simulink model "guidance_fuzzy_alt"  (R2017b)
settings: Solver=FixedStepDiscrete  StartTime=0.0  StopTime=inf  FixedStep=0.01  RelTol=1e-3
model workspace (MAT data in the model file):
  SL_ROS_VariableLengthArrays_MaxSizes.CommonInfo.ArrayTruncateAction = 'EmitWarning'
  SL_ROS_VariableLengthArrays_MaxSizes.MsgTypeMap = containers.Map
  SL_ROS_VariableLengthArrays_MaxSizes.MsgTypeMap.serialization.keys = {'sensor_msgs/Image'}
  SL_ROS_VariableLengthArrays_MaxSizes.MsgTypeMap.serialization.values{1}(1).PropertyName = 'Encoding'
  SL_ROS_VariableLengthArrays_MaxSizes.MsgTypeMap.serialization.values{1}(1).DataType = 'uint8'
  SL_ROS_VariableLengthArrays_MaxSizes.MsgTypeMap.serialization.values{1}(1).MaxLength = 128
  SL_ROS_VariableLengthArrays_MaxSizes.MsgTypeMap.serialization.values{1}(2).PropertyName = 'Data'
  SL_ROS_VariableLengthArrays_MaxSizes.MsgTypeMap.serialization.values{1}(2).DataType = 'uint8'
  SL_ROS_VariableLengthArrays_MaxSizes.MsgTypeMap.serialization.values{1}(2).MaxLength = 921600
  SL_ROS_VariableLengthArrays_MaxSizes.MsgTypeMap.serialization.uniformity = 0
  SL_ROS_VariableLengthArrays_MaxSizes.MsgTypeMap.serialization.keyType = 'char'
  SL_ROS_VariableLengthArrays_MaxSizes.MsgTypeMap.serialization.valueType = 'any'
undefined symbols (not defined in the file): Data, Data_SL_Info
libraries: dspstat3 x14, robotlib x10, simulink_extras x7, simulink x4, dspswit3 x1
(part 1 of 2)
settings Model: SimulationMode=external  Creator=a  LastModifiedBy=Alien
settings OptimizationCC: MaxStackSize=64
settings DebuggingCC: ParameterTunabilityLossMsg=error
settings HardwareCC: ProdBitPerPointer=32  ProdBitPerSizeT=32  ProdBitPerPtrDiffT=32  ProdLargestAtomicInteger=Long  ProdLargestAtomicFloat=Double  ProdWordSize=32  ProdHWDeviceType=ARM Compatible->ARM Cortex
settings SFSimCC: MATLABDynamicMemAlloc=off
settings RTWCC: SystemTargetFile=ert.tlc  HardwareBoard=Robot Operating System (ROS)  TemplateMakefile=ert_default_tmf  GenerateReport=on  Toolchain=Catkin  IncludeHyperlinkInReport=on  LaunchReport=on  TargetLang=C++  GenerateTraceInfo=on  GenerateTraceReport=on  GenerateTraceReportSl=on  GenerateTraceReportSf=on  GenerateTraceReportEml=on
settings CodeAppCC: ForceParamTrailComments=on  IgnoreCustomStorageClasses=off  OperatorAnnotations=on  SimulinkDataObjDesc=on  SFDataObjDesc=on  MATLABFcnDesc=on  InsertBlockDesc=on  StateflowObjectComments=on  MATLABSourceComments=on
settings ERTTargetCC: MultiwordLength=2048  ExtMode=on  ExtModeMexArgs='192.168.2.2' 0 17725
settings SimscapeCC: SimscapeNormalizeSystem=off

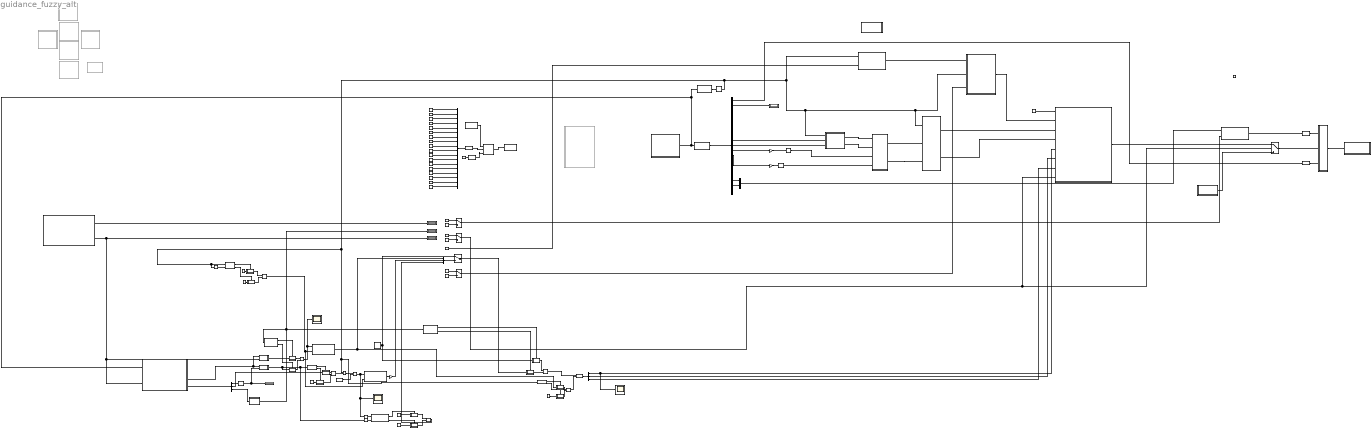
== system guidance_fuzzy_alt ==
  note: Subsystem
  Abs6 : Abs
  Abs7 : Abs
  Assignment : Assignment  DiagnosticForDimensions=Warning  IndexOptions=Index vector (dialog)  Indices=1  OutputSizes=1
  Blank Message : robotlib/Blank Message  SourceLibraryInfo=This block requires Robotics System Toolbox  messageType=std_msgs/UInt8MultiArray  SampleTime=inf
      settings: SourceProductBaseCode=RO
  Bus Assignment : BusAssignment  AssignedSignals=Data,Data_SL_Info.CurrentLength
  Constant : Constant  Value=[0 0 0]
  Constant1 : Constant  Value=18:128
  Constant2 : Constant  Value=0
  Constant3 : Constant  Value=17
  Constant4 : Constant
  Constant5 : Constant  Value=0
  Constant6 : Constant  Value=0
  "Count_QRcodes " : Display
  Course : Display
  Data Store Memory : DataStoreMemory  DataStoreName=kill  ReadBeforeWriteMsg=warning  WriteAfterWriteMsg=warning  WriteAfterReadMsg=warning  ShowAdditionalParam=off
  Data Type Conversion18 : DataTypeConversion  OutDataTypeStr=uint8
  Data Type Conversion19 : DataTypeConversion  OutDataTypeStr=uint32
  Data Type Conversion3 : DataTypeConversion  OutDataTypeStr=single
  Data Type Conversion4 : DataTypeConversion  OutDataTypeStr=single
  DataChangeTimer : Subsystem
  Demux : Demux  Outputs=19
  Demux1 : Demux  Outputs=3
  Demux6 : Demux  Outputs=3
  Discrete PID Controller : simulink/Continuous/PID Controller  Controller=PID  TimeDomain=Discrete-time  SampleTime=-1  IntegratorMethod=Forward Euler  FilterMethod=Forward Euler  Form=Parallel  UseFilter=on  ControllerParametersSource=internal  P=0.4  I=0.001  D=0  N=100  InitialConditionSource=internal  InitialConditionForIntegrator=0  InitialConditionForFilter=0  ExternalReset=either  LimitOutput=on  UpperSaturationLimit=10  LowerSaturationLimit=-10  LinearizeAsGain=off  AntiWindupMode=none  Kb=1  TrackingMode=off  Kt=1  PParamMin=[]  PParamMax=[]  IParamMin=[]  IParamMax=[]  DParamMin=[]  DParamMax=[]  NParamMin=[]  NParamMax=[]  KbParamMin=[]  KbParamMax=[]  KtParamMin=[]  KtParamMax=[]  POutMin=[]  POutMax=[]  IOutMin=[]  IOutMax=[]  DOutMin=[]  DOutMax=[]  NOutMin=[]  NOutMax=[]  KbOutMin=[]  KbOutMax=[]  KtOutMin=[]  KtOutMax=[]  IntegratorOutMin=[]  IntegratorOutMax=[]  FilterOutMin=[]  FilterOutMax=[]  SumOutMin=[]  SumOutMax=[]  SumI1OutMin=[]  SumI1OutMax=[]  SumI2OutMin=[]  SumI2OutMax=[]  SumI3OutMin=[]  SumI3OutMax=[]  SumDOutMin=[]  SumDOutMax=[]  SaturationOutMin=[]  SaturationOutMax=[]  IntegratorContinuousStateAttributes=''  IntegratorStateMustResolveToSignalObject=off  IntegratorRTWStateStorageClass=Auto  FilterContinuousStateAttributes=''  FilterStateMustResolveToSignalObject=off  FilterRTWStateStorageClass=Auto  DifferentiatorICPrevScaledInput=0  DifferentiatorOutMin=[]  DifferentiatorOutMax=[]  InitialConditionSetting=State (most efficient)  FilterDiffOutCoefMin=[]  FilterDiffOutCoefMax=[]  SumDenOutMin=[]  SumDenOutMax=[]  SumNumOutMin=[]  SumNumOutMax=[]  ReciprocalOutMin=[]  ReciprocalOutMax=[]  DivideOutMin=[]  DivideOutMax=[]  TunerSelectOption=Transfer Function Based (PID Tuner App)
  Discrete PID Controller1 : simulink/Continuous/PID Controller  Controller=PID  TimeDomain=Discrete-time  SampleTime=-1  IntegratorMethod=Forward Euler  FilterMethod=Forward Euler  Form=Parallel  UseFilter=on  ControllerParametersSource=internal  P=0.2  I=0  D=0  N=100  InitialConditionSource=internal  InitialConditionForIntegrator=0  InitialConditionForFilter=0  ExternalReset=either  LimitOutput=on  UpperSaturationLimit=0.5  LowerSaturationLimit=-0.5  LinearizeAsGain=off  AntiWindupMode=none  Kb=1  TrackingMode=off  Kt=1  PParamMin=[]  PParamMax=[]  IParamMin=[]  IParamMax=[]  DParamMin=[]  DParamMax=[]  NParamMin=[]  NParamMax=[]  KbParamMin=[]  KbParamMax=[]  KtParamMin=[]  KtParamMax=[]  POutMin=[]  POutMax=[]  IOutMin=[]  IOutMax=[]  DOutMin=[]  DOutMax=[]  NOutMin=[]  NOutMax=[]  KbOutMin=[]  KbOutMax=[]  KtOutMin=[]  KtOutMax=[]  IntegratorOutMin=[]  IntegratorOutMax=[]  FilterOutMin=[]  FilterOutMax=[]  SumOutMin=[]  SumOutMax=[]  SumI1OutMin=[]  SumI1OutMax=[]  SumI2OutMin=[]  SumI2OutMax=[]  SumI3OutMin=[]  SumI3OutMax=[]  SumDOutMin=[]  SumDOutMax=[]  SaturationOutMin=[]  SaturationOutMax=[]  IntegratorContinuousStateAttributes=''  IntegratorStateMustResolveToSignalObject=off  IntegratorRTWStateStorageClass=Auto  FilterContinuousStateAttributes=''  FilterStateMustResolveToSignalObject=off  FilterRTWStateStorageClass=Auto  DifferentiatorICPrevScaledInput=0  DifferentiatorOutMin=[]  DifferentiatorOutMax=[]  InitialConditionSetting=State (most efficient)  FilterDiffOutCoefMin=[]  FilterDiffOutCoefMax=[]  SumDenOutMin=[]  SumDenOutMax=[]  SumNumOutMin=[]  SumNumOutMax=[]  ReciprocalOutMin=[]  ReciprocalOutMax=[]  DivideOutMin=[]  DivideOutMax=[]  TunerSelectOption=Transfer Function Based (PID Tuner App)
  Display10 : Display
  Divide : Product  Inputs=*/
  Gain2 : Gain  Gain=-1
  If : If  NumInputs=2  IfExpression=u1 < 0.15 & u2 < 15
  If Action Subsystem : Subsystem  TreatAsAtomicUnit=on
  If Action Subsystem1 : Subsystem  TreatAsAtomicUnit=on
  If Action Subsystem10 : Subsystem  TreatAsAtomicUnit=on
  If Action Subsystem11 : Subsystem  TreatAsAtomicUnit=on
  If Action Subsystem2 : Subsystem  TreatAsAtomicUnit=on
  If Action Subsystem3 : Subsystem  TreatAsAtomicUnit=on
  If Action Subsystem4 : Subsystem  TreatAsAtomicUnit=on
  If Action Subsystem5 : Subsystem  TreatAsAtomicUnit=on
  If Action Subsystem6 : Subsystem  TreatAsAtomicUnit=on
  If Action Subsystem7 : Subsystem  TreatAsAtomicUnit=on
  If Action Subsystem8 : Subsystem  TreatAsAtomicUnit=on
  If Action Subsystem9 : Subsystem  TreatAsAtomicUnit=on
  If1 : If  IfExpression=u1 < 10
  If11 : If  IfExpression=u1 > 2
  If2 : If  IfExpression=u1 > 2
  If3 : If  NumInputs=2  IfExpression=u1 > 0.2 & u2<0.2
  If4 : If  IfExpression=u1 > 0.2
  Manual Switch : ManualSwitch
  Memory : Memory
  Merge{,1..5} (6 alike) : Merge
  Moving Average : dspstat3/Moving Average  Method=Sliding window  SpecifyWindowLength=on  WindowLength=30  ForgettingFactor=0.9  SimulateUsing=Code generation
  Mux3 : Mux  Inputs=3
  Mux4 : Mux  Inputs=2
  Mux8 : Mux  Inputs=18
  P Moving Average : dspstat3/Moving Average  Method=Sliding window  SpecifyWindowLength=on  WindowLength=35  ForgettingFactor=0.9  SimulateUsing=Code generation
  Product : Product
  Publish : robotlib/Publish  SourceLibraryInfo=This block requires Robotics System Toolbox  topicSource=Specify your own  topic=/quadrotor_1/params  messageType=std_msgs/UInt8MultiArray  messageQueueLength=1
      settings: SourceProductBaseCode=RO
  Push Button : Subsystem  Commented=on  DialogController=hmiCreateDDGDialog  IsWebBlock=on  mask(MWDashboardBlock){webBlockId=dc87a16a-ce0b-429d-b1f9-30aaadb48afa, webBlockType=pushbutton, ShowInLibBrwoser=on, ShowInitialText=on, HMISrcModelName=guidance_fuzzy_alt}
      mask prompts: webBlockId "WebBlock Id"; webBlockType "WebBlock Type"; HMISrcModelName "Source Model"
      mask help: SimulinkHMI:dialogs:PushButtonDialogDesc
      mask Help: helpview([docroot '/mapfiles/simulink.map'], 'hmi_push_button')
      mask Display:
      | model = bdroot(gcb);
      | if strcmp(get_param(model,'BlockDiagramType'), 'library')
      |     image([(matlabroot) '/toolbox/simulink/hmi/icons/PushButton.png']);
      | end
  Push Button1 : Subsystem  Commented=on  DialogController=hmiCreateDDGDialog  IsWebBlock=on  mask(MWDashboardBlock){webBlockId=24acbbf4-6844-475c-bdac-e05cc7a3fcf0, webBlockType=pushbutton, ShowInLibBrwoser=on, ShowInitialText=on, HMISrcModelName=guidance_fuzzy_alt}
      mask prompts: webBlockId "WebBlock Id"; webBlockType "WebBlock Type"; HMISrcModelName "Source Model"
      mask help: SimulinkHMI:dialogs:PushButtonDialogDesc
      mask Help: helpview([docroot '/mapfiles/simulink.map'], 'hmi_push_button')
      mask Display:
      | model = bdroot(gcb);
      | if strcmp(get_param(model,'BlockDiagramType'), 'library')
      |     image([(matlabroot) '/toolbox/simulink/hmi/icons/PushButton.png']);
      | end
  Push Button2 : Subsystem  Commented=on  DialogController=hmiCreateDDGDialog  IsWebBlock=on  mask(MWDashboardBlock){webBlockId=70708495-3a8b-4125-b41c-8b8a1e915131, webBlockType=pushbutton, ShowInLibBrwoser=on, ShowInitialText=on, HMISrcModelName=guidance_fuzzy_alt}
      mask prompts: webBlockId "WebBlock Id"; webBlockType "WebBlock Type"; HMISrcModelName "Source Model"
      mask help: SimulinkHMI:dialogs:PushButtonDialogDesc
      mask Help: helpview([docroot '/mapfiles/simulink.map'], 'hmi_push_button')
      mask Display:
      | model = bdroot(gcb);
      | if strcmp(get_param(model,'BlockDiagramType'), 'library')
      |     image([(matlabroot) '/toolbox/simulink/hmi/icons/PushButton.png']);
      | end
  Push Button3 : Subsystem  Commented=on  DialogController=hmiCreateDDGDialog  IsWebBlock=on  mask(MWDashboardBlock){webBlockId=ffc355a9-f3f0-46c2-899e-34688d84451c, webBlockType=pushbutton, ShowInLibBrwoser=on, ShowInitialText=on, HMISrcModelName=guidance_fuzzy_alt}
      mask prompts: webBlockId "WebBlock Id"; webBlockType "WebBlock Type"; HMISrcModelName "Source Model"
      mask help: SimulinkHMI:dialogs:PushButtonDialogDesc
      mask Help: helpview([docroot '/mapfiles/simulink.map'], 'hmi_push_button')
      mask Display:
      | model = bdroot(gcb);
      | if strcmp(get_param(model,'BlockDiagramType'), 'library')
      |     image([(matlabroot) '/toolbox/simulink/hmi/icons/PushButton.png']);
      | end
  Push Button4 : Subsystem  Commented=on  DialogController=hmiCreateDDGDialog  IsWebBlock=on  mask(MWDashboardBlock){webBlockId=54db0c4f-5f86-4b76-bb6a-5be3d8ea16bb, webBlockType=pushbutton, ShowInLibBrwoser=on, ShowInitialText=on, HMISrcModelName=guidance_fuzzy_alt}
      mask prompts: webBlockId "WebBlock Id"; webBlockType "WebBlock Type"; HMISrcModelName "Source Model"
      mask help: SimulinkHMI:dialogs:PushButtonDialogDesc
      mask Help: helpview([docroot '/mapfiles/simulink.map'], 'hmi_push_button')
      mask Display:
      | model = bdroot(gcb);
      | if strcmp(get_param(model,'BlockDiagramType'), 'library')
      |     image([(matlabroot) '/toolbox/simulink/hmi/icons/PushButton.png']);
      | end
  Push Button5 : Subsystem  Commented=on  DialogController=hmiCreateDDGDialog  IsWebBlock=on  mask(MWDashboardBlock){webBlockId=7ebe0749-6d9c-49fd-940b-537e52e049aa, webBlockType=pushbutton, ShowInLibBrwoser=on, ShowInitialText=on, HMISrcModelName=guidance_fuzzy_alt}
      mask prompts: webBlockId "WebBlock Id"; webBlockType "WebBlock Type"; HMISrcModelName "Source Model"
      mask help: SimulinkHMI:dialogs:PushButtonDialogDesc
      mask Help: helpview([docroot '/mapfiles/simulink.map'], 'hmi_push_button')
      mask Display:
      | model = bdroot(gcb);
      | if strcmp(get_param(model,'BlockDiagramType'), 'library')
      |     image([(matlabroot) '/toolbox/simulink/hmi/icons/PushButton.png']);
      | end
  Q Moving Average : dspstat3/Moving Average  Method=Sliding window  SpecifyWindowLength=on  WindowLength=35  ForgettingFactor=0.9  SimulateUsing=Code generation
  Scope1 : Scope
  Scope2 : Scope
  Scope3 : Scope
  Selector : Selector  InputPortWidth=26  IndexOptions=Index vector (dialog)  Indices=[17:26 4 5 6 11 12 13 1:3]  OutputSizes=1
  Selector1 : Selector  InputPortWidth=26  IndexOptions=Index vector (dialog)  Indices=[7]  OutputSizes=1
  Slider Switch : Subsystem  Commented=on  DialogController=hmiCreateDDGDialog  IsWebBlock=on  mask(MWDashboardBlock){webBlockId=a556c2db-78b9-4d66-bd76-d44e139280cd, webBlockType=sliderswitch, ShowInLibBrowser=on, ShowInitialText=on, HMISrcModelName=guidance_fuzzy_alt}
      mask prompts: webBlockId "WebBlock Id"; webBlockType "WebBlock Type"; HMISrcModelName "Source Model"
      mask help: SimulinkHMI:dialogs:SwitchDialogDesc
      mask Help: helpview([docroot '/mapfiles/simulink.map'], 'hmi_slider_switch')
      mask Display:
      | if strcmp(get_param(bdroot(gcb),'BlockDiagramType'), 'library')
      |     image([(matlabroot) '/toolbox/simulink/hmi/icons/SliderSwitch.png']);
      | end
  Sonar Moving Average : dspstat3/Moving Average  Method=Sliding window  SpecifyWindowLength=on  WindowLength=5  ForgettingFactor=0.9  SimulateUsing=Code generation
  Subsystem : Subsystem
  Subsystem2 : Subsystem
  Subsystem5 : Subsystem
  Subsystem6 : Subsystem
  Switch : Switch  Criteria=u2 > Threshold
  "TIme_From Last_line " : Display
  approx_poly_eppsilon_coef : Constant  Value=2
  arm_switch : ManualSwitch
  aspect_ratio_max : Constant  Value=100
  aspect_ratio_min : Constant  Value=3
  attitude_failsafe : Subsystem
  camera_trigonometric_factor(m/pix) : Constant  Value=342.85
  check_arm_status : Subsystem
  command_input : Subsystem  Commented=on
  command_output : Subsystem
  compensate_angular_velocity_effect_on_of : Subsystem
  corrupt_max_area : Constant  Value=60
  "dark_max_b " : Constant  Value=90
  dark_max_g : Constant  Value=90
  dark_max_r : Constant  Value=90
  dark_min_b : Constant  Value=0
  dark_min_g : Constant  Value=0
  dark_min_r : Constant  Value=0
  "data_input " : Subsystem
  land : ManualSwitch
  manual_control : Subsystem  mask{throttle=0.0, roll=0, pitch=0, yaw=0, mode=2}
  manual_throttle : Subsystem  mask{th=90}
  max_diviation : Constant  Value=40
  mode : Constant  Value=2
  movement_velocity : Constant  Value=0.1
  movement_velocity1 : Constant  Value=0
  one : Constant
  one1 : Constant
  one2 : Constant
  optimize_error_psi(deg)1 : Subsystem
  optimize_error_psi(deg)3 : Subsystem
  p gain : Gain  Gain=3.1415 / 180.0
  pixel_per_sec_to_m_per_sec : Subsystem
  q gain : Gain  Gain=3.1415 / 180.0
  radio_command_frame_rate : Display
  take_off_switch : ManualSwitch
  throttle_handler_climb_mode : Subsystem
  velocity_control : Subsystem
  white_max_b : Constant  Value=255
  white_max_g : Constant  Value=255
  white_max_r : Constant  Value=255
  white_min_b : Constant  Value=120
  white_min_g : Constant  Value=120
  white_min_r : Constant  Value=120
  z_des : Constant
  zero : Constant  Value=0
  zero1 : Constant  Value=0
  zero2 : Constant  Value=0
  wires:
  check_arm_status/1(Out) -> command_output/1(command)
  Data Type Conversion3/1 -> check_arm_status/3(motors_on)
  Data Type Conversion4/1 -> check_arm_status/1(arm)
  manual_control/1(commands) -> Switch/3
  Switch/1 -> check_arm_status/2(command)
  Selector/1 -> Demux/1
  Demux/1 -> Data Type Conversion3/1
  Demux/2 -> radio_command_frame_rate/1
  mode/1 -> velocity_control/1(mode)
  Selector1/1 -> Sonar Moving Average/1
  velocity_control/1(radio_command) -> Switch/1
  Sonar Moving Average/1 -> Memory/1, If3/1, If4/1, Product/1, pixel_per_sec_to_m_per_sec/1(height), Subsystem5/1(height), throttle_handler_climb_mode/2(height), Subsystem2/1(measured_height)
  Demux/11 -> p gain/1
  Demux/12 -> q gain/1
  p gain/1 -> P Moving Average/1
  q gain/1 -> Q Moving Average/1
  Demux/9 -> pixel_per_sec_to_m_per_sec/2(vx(pix/sec))
  Demux/10 -> pixel_per_sec_to_m_per_sec/3(vy(pix/sec))
  throttle_handler_climb_mode/1(throttle) -> velocity_control/2(throttle)
  pixel_per_sec_to_m_per_sec/1(vx(m/s)) -> compensate_angular_velocity_effect_on_of/1(vx)
  pixel_per_sec_to_m_per_sec/2(vy(m/s)) -> compensate_angular_velocity_effect_on_of/2(vy)
  P Moving Average/1 -> compensate_angular_velocity_effect_on_of/3(p)
  Q Moving Average/1 -> compensate_angular_velocity_effect_on_of/4(q)
  compensate_angular_velocity_effect_on_of/1(corrected_vx) -> Subsystem5/2(vx)
  compensate_angular_velocity_effect_on_of/2(corrected_vy) -> Subsystem5/3(vy)
  Subsystem5/1(vx_out) -> velocity_control/3(vx)
  Subsystem5/2(vy_out) -> velocity_control/4(vy)
  Subsystem2/1(throttle_command) -> throttle_handler_climb_mode/1(desired_throttle)
  Demux6/1 -> Scope3/1, velocity_control/5(yaw_des_rate)
  Demux6/2 -> velocity_control/6(vy_setpoint)
  If1/2 -> If Action Subsystem3/Action
  "data_input "/1(data) -> Subsystem6/1(In1), Selector1/1, Selector/1
  Demux1/1 -> Moving Average/1
  If Action Subsystem3/1(Out1) -> Merge1/2
  optimize_error_psi(deg)3/1(Out1) -> If Action Subsystem4/1(In1), Abs7/1, If1/1
  Constant2/1 -> If Action Subsystem3/1(In1)
  Discrete PID Controller1/1 -> Gain2/1
  Product/1 -> Divide/1
  camera_trigonometric_factor(m/pix)/1 -> Divide/2
  Divide/1 -> Scope2/1, Abs6/1, Discrete PID Controller1/1
  Demux1/2 -> If Action Subsystem2/1(In1)
  If1/1 -> If Action Subsystem2/Action
  Merge1/1 -> Product/2
  Moving Average/1 -> Display10/1, optimize_error_psi(deg)3/2(psi1)
  If Action Subsystem2/1(Out1) -> Merge1/1
  Demux/17 -> Mux4/1
  Demux/18 -> Mux4/2
  Mux4/1 -> attitude_failsafe/1(attitude)
  Demux1/3 -> DataChangeTimer/1(trig)
  attitude_failsafe/1(arm_command) -> Data Type Conversion4/1
  Abs6/1 -> If/1
  Abs7/1 -> If/2
  If/1 -> If Action Subsystem/Action
  If/2 -> If Action Subsystem6/Action
  movement_velocity/1 -> If Action Subsystem/1(In1)
  movement_velocity1/1 -> If Action Subsystem6/1(In1)
  If Action Subsystem/1(Out1) -> Merge/1
  If Action Subsystem6/1(Out1) -> Merge/2
  Demux6/3 -> velocity_control/7(vx_setpoint)
  If11/2 -> If Action Subsystem7/Action
  If Action Subsystem7/1(Out1) -> Merge2/2
  If11/1 -> If Action Subsystem8/Action
  If Action Subsystem8/1(Out1) -> Merge2/1
  Merge2/1 -> Assignment/1
  white_max_r/1 -> Mux8/12
  Mux8/1 -> Data Type Conversion18/1
  dark_max_r/1 -> Mux8/6
  dark_min_r/1 -> Mux8/3
  white_max_g/1 -> Mux8/11
  approx_poly_eppsilon_coef/1 -> Mux8/16
  aspect_ratio_min/1 -> Mux8/14
  white_max_b/1 -> Mux8/10
  white_min_g/1 -> Mux8/8
  aspect_ratio_max/1 -> Mux8/13
  white_min_b/1 -> Mux8/7
  Bus Assignment/1 -> Publish/1
  max_diviation/1 -> Mux8/15
  dark_max_g/1 -> Mux8/5
  dark_min_b/1 -> Mux8/1
  Blank Message/1 -> Bus Assignment/1
  Constant1/1 -> Mux8/18
  dark_min_g/1 -> Mux8/2
  Data Type Conversion18/1 -> Bus Assignment/2
  Constant3/1 -> Data Type Conversion19/1
  "dark_max_b "/1 -> Mux8/4
  white_min_r/1 -> Mux8/9
  corrupt_max_area/1 -> Mux8/17
  Data Type Conversion19/1 -> Bus Assignment/3
  take_off_switch/1 -> Switch/2, velocity_control/8(Integrator_reset)
  z_des/1 -> Subsystem2/2(z_desired)
  land/1 -> throttle_handler_climb_mode/3(landing)
  arm_switch/1 -> attitude_failsafe/2(user_arm_command)
  Manual Switch/1 -> If Action Subsystem7/1(In1)
  DataChangeTimer/1(diff_time) -> If2/1, "TIme_From Last_line "/1, If11/1
  Gain2/1 -> Mux3/2
  zero2/1 -> land/1
  one/1 -> arm_switch/2
  zero/1 -> arm_switch/1
  Discrete PID Controller/1 -> If Action Subsystem10/1(In1), Mux3/1
  Constant/1 -> Manual Switch/1, If Action Subsystem8/1(In1)
  Mux3/1 -> Manual Switch/2
  one1/1 -> take_off_switch/2
  zero1/1 -> take_off_switch/1
  one2/1 -> land/2
  Merge/1 -> Mux3/3
  Subsystem/2(Out4) -> Course/1, optimize_error_psi(deg)1/2(psi1), Subsystem6/2(In2)
  Subsystem/1(Out3) -> "Count_QRcodes "/1
  Subsystem6/3(Out3) -> optimize_error_psi(deg)1/1(psi2), optimize_error_psi(deg)3/1(psi2)
  Subsystem6/4(Out4) -> Demux1/1
  If2/1 -> If Action Subsystem1/Action
  optimize_error_psi(deg)1/1(Out1) -> If Action Subsystem1/1(In1)
  If2/2 -> If Action Subsystem4/Action
  If Action Subsystem1/1(Out1) -> Merge3/1
  If Action Subsystem4/1(Out1) -> Merge3/2
  Merge3/1 -> Scope1/1, Discrete PID Controller/1
  Memory/1 -> If3/2
  If3/1 -> If Action Subsystem5/Action
  If3/2 -> If Action Subsystem9/Action
  Constant4/1 -> If Action Subsystem5/1(In1)
  Constant5/1 -> If Action Subsystem9/1(In1)
  If Action Subsystem5/1(Out1) -> Merge4/1
  If Action Subsystem9/1(Out1) -> Merge4/2
  Merge4/1 -> Discrete PID Controller1/2, Discrete PID Controller/2
  Assignment/1 -> Demux6/1
  If4/1 -> If Action Subsystem10/Action
  If4/2 -> If Action Subsystem11/Action
  Constant6/1 -> If Action Subsystem11/1(In1)
  If Action Subsystem10/1(Out1) -> Merge5/1
  If Action Subsystem11/1(Out1) -> Merge5/2
  Merge5/1 -> Assignment/2

== system guidance_fuzzy_alt/DataChangeTimer ==
  trig : Inport
  Abs : Abs
  Data Type Conversion : DataTypeConversion  OutDataTypeStr=uint8
  Digital Clock : DigitalClock  SampleTime=0.01
  If : If
  If Action Subsystem : Subsystem  TreatAsAtomicUnit=on
  If Action Subsystem1 : Subsystem  TreatAsAtomicUnit=on
  Subtract : Sum  Inputs=+-
  diff_time : Outport
  wires:
  If Action Subsystem1/1(Out1) -> Subtract/2
  Subtract/1 -> Abs/1
  trig/1 -> Data Type Conversion/1
  Abs/1 -> diff_time/1
  If Action Subsystem/1(Out1) -> Subtract/1
  Digital Clock/1 -> If Action Subsystem1/1(In1), If Action Subsystem/1(In1)
  If/2 -> If Action Subsystem1/Action
  If/1 -> If Action Subsystem/Action
  Data Type Conversion/1 -> If/1

== system guidance_fuzzy_alt/If Action Subsystem ==
  In1 : Inport
  Action Port : ActionPort  ActionType=then
  Out1 : Outport
  wires:
  In1/1 -> Out1/1

== system guidance_fuzzy_alt/If Action Subsystem1 ==
  In1 : Inport
  Action Port : ActionPort  ActionType=then
  Out1 : Outport
  wires:
  In1/1 -> Out1/1

== system guidance_fuzzy_alt/If Action Subsystem10 ==
  In1 : Inport
  Action Port : ActionPort  ActionType=then
  Out1 : Outport
  wires:
  In1/1 -> Out1/1

== system guidance_fuzzy_alt/If Action Subsystem11 ==
  In1 : Inport
  Action Port : ActionPort  ActionType=else
  Out1 : Outport
  wires:
  In1/1 -> Out1/1

== system guidance_fuzzy_alt/If Action Subsystem2 ==
  In1 : Inport
  Action Port : ActionPort  ActionType=then
  Out1 : Outport
  wires:
  In1/1 -> Out1/1

== system guidance_fuzzy_alt/If Action Subsystem3 ==
  In1 : Inport
  Action Port : ActionPort  ActionType=else
  Out1 : Outport
  wires:
  In1/1 -> Out1/1

== system guidance_fuzzy_alt/If Action Subsystem4 ==
  In1 : Inport
  Action Port : ActionPort  ActionType=else
  Out1 : Outport
  wires:
  In1/1 -> Out1/1

== system guidance_fuzzy_alt/If Action Subsystem5 ==
  In1 : Inport
  Action Port : ActionPort  ActionType=then
  Out1 : Outport
  wires:
  In1/1 -> Out1/1

== system guidance_fuzzy_alt/If Action Subsystem6 ==
  In1 : Inport
  Action Port : ActionPort  ActionType=else
  Out1 : Outport
  wires:
  In1/1 -> Out1/1

== system guidance_fuzzy_alt/If Action Subsystem7 ==
  In1 : Inport
  Action Port : ActionPort  ActionType=else
  Out1 : Outport
  wires:
  In1/1 -> Out1/1

== system guidance_fuzzy_alt/If Action Subsystem8 ==
  In1 : Inport
  Action Port : ActionPort  ActionType=then
  Out1 : Outport
  wires:
  In1/1 -> Out1/1

== system guidance_fuzzy_alt/If Action Subsystem9 ==
  In1 : Inport
  Action Port : ActionPort  ActionType=else
  Out1 : Outport
  wires:
  In1/1 -> Out1/1

== system guidance_fuzzy_alt/Push Button ==

== system guidance_fuzzy_alt/Push Button1 ==

== system guidance_fuzzy_alt/Push Button2 ==

== system guidance_fuzzy_alt/Push Button3 ==

== system guidance_fuzzy_alt/Push Button4 ==

== system guidance_fuzzy_alt/Push Button5 ==

== system guidance_fuzzy_alt/Slider Switch ==

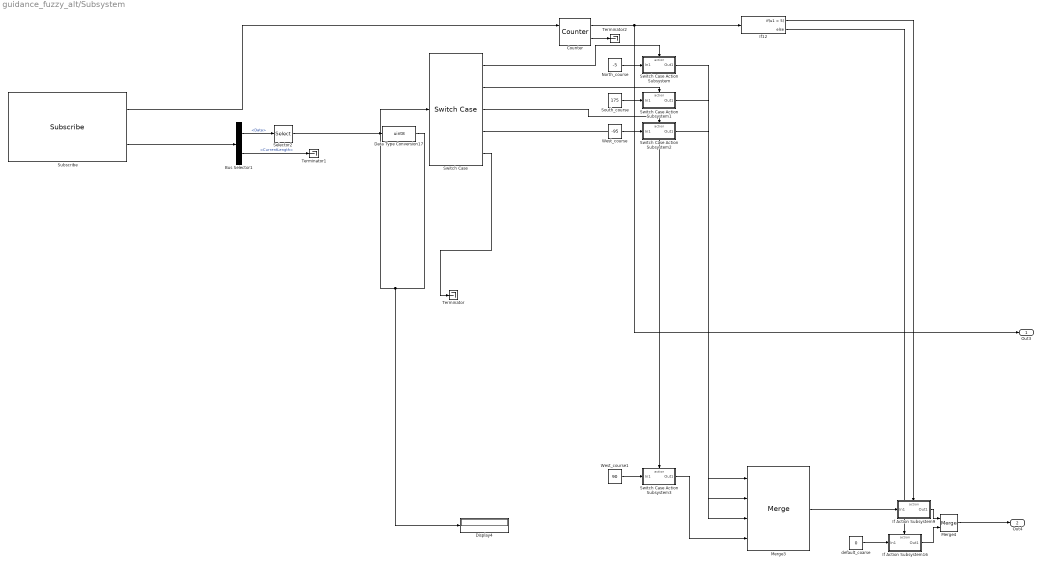
== system guidance_fuzzy_alt/Subsystem ==
  Bus Selector1 : BusSelector  OutputSignals=Data,Data_SL_Info.CurrentLength
  Counter : dspswit3/Counter  Direction=Up  CountEvent=Rising edge  CounterSize=User defined  MaxCount=1000000  InitialCount=0  Output=Count and Hit  HitValue=10  ResetInput=on  SamplesPerFrame=1  Ts=1  CntDtype=double  HitDtype=Logical
  Data Type Conversion17 : DataTypeConversion  OutDataTypeStr=uint8
  Display4 : Display
  If Action Subsystem16 : Subsystem  TreatAsAtomicUnit=on
  If Action Subsystem9 : Subsystem  TreatAsAtomicUnit=on
  If12 : If  IfExpression=u1 > 5
  Merge3 : Merge  Inputs=4
  Merge4 : Merge
  North_course : Constant  Value=-5
  Selector2 : Selector  InputPortWidth=128  IndexOptions=Index vector (dialog)  Indices=[1]  OutputSizes=1
  South_course : Constant  Value=175
  Subscribe : robotlib/Subscribe  SourceLibraryInfo=This block requires Robotics System Toolbox  topicSource=Select from ROS network  topic=/quadrotor_1/qr_data  messageType=std_msgs/String  sampleTime=-1  messageQueueLength=1
      settings: SourceProductBaseCode=RO
  Switch Case : SwitchCase  CaseConditions="{78, 83, 87,  69}"
  Switch Case Action Subsystem : Subsystem  TreatAsAtomicUnit=on
  Switch Case Action Subsystem1 : Subsystem  TreatAsAtomicUnit=on
  Switch Case Action Subsystem2 : Subsystem  TreatAsAtomicUnit=on
  Switch Case Action Subsystem3 : Subsystem  TreatAsAtomicUnit=on
  Terminator : Terminator
  Terminator1 : Terminator
  Terminator2 : Terminator
  West_course : Constant  Value=-95
  West_course1 : Constant  Value=90
  default_coarse : Constant  Value=0
  Out3 : Outport
  Out4 : Outport  Port=2
  wires:
  Counter/1 -> Out3/1, If12/1
  Merge4/1 -> Out4/1
  Counter/2 -> Terminator2/1
  If Action Subsystem16/1(Out1) -> Merge4/2
  If12/2 -> If Action Subsystem16/Action
  Bus Selector1/1 -> Selector2/1  "<Data>"
  Subscribe/2 -> Bus Selector1/1
  Switch Case/3 -> Switch Case Action Subsystem2/Action
  Switch Case/2 -> Switch Case Action Subsystem1/Action
  South_course/1 -> Switch Case Action Subsystem1/1(In1)
  West_course/1 -> Switch Case Action Subsystem2/1(In1)
  West_course1/1 -> Switch Case Action Subsystem3/1(In1)
  Switch Case/4 -> Switch Case Action Subsystem3/Action
  Switch Case/5 -> Terminator/1
  Switch Case Action Subsystem1/1(Out1) -> Merge3/2
  Switch Case Action Subsystem/1(Out1) -> Merge3/1
  Switch Case Action Subsystem2/1(Out1) -> Merge3/3
  Subscribe/1 -> Counter/1
  Switch Case Action Subsystem3/1(Out1) -> Merge3/4
  If12/1 -> If Action Subsystem9/Action
  Merge3/1 -> If Action Subsystem9/1(In1)
  If Action Subsystem9/1(Out1) -> Merge4/1
  default_coarse/1 -> If Action Subsystem16/1(In1)
  North_course/1 -> Switch Case Action Subsystem/1(In1)
  Switch Case/1 -> Switch Case Action Subsystem/Action
  Selector2/1 -> Data Type Conversion17/1
  Data Type Conversion17/1 -> Switch Case/1, Display4/1
  Bus Selector1/2 -> Terminator1/1  "<CurrentLength>"

== system guidance_fuzzy_alt/Subsystem2 ==
  measured_height : Inport
  z_desired : Inport  Port=2
  Constant : Constant  Value=68
  Constant1 : Constant  Value=40
  Constant2 : Constant  Value=50
  Data Type Conversion : DataTypeConversion  OutDataTypeStr=single
  If : If  IfExpression=u1 > 0.15  ElseIfExpressions=u1 < -0.15
  If Action Subsystem : Subsystem  TreatAsAtomicUnit=on
  If Action Subsystem1 : Subsystem  TreatAsAtomicUnit=on
  If Action Subsystem2 : Subsystem  TreatAsAtomicUnit=on
  Merge : Merge  Inputs=3
  Moving Average : dspstat3/Moving Average  Method=Sliding window  SpecifyWindowLength=on  WindowLength=60  ForgettingFactor=0.9  SimulateUsing=Code generation
  Sum2 : Sum  Inputs=|+-
  To Workspace : ToWorkspace  VariableName=simout  SaveFormat=Timeseries  SampleTime=-1
  To Workspace1 : ToWorkspace  VariableName=simout1  SaveFormat=Timeseries  SampleTime=-1
  Z_command : Scope
  Z_error : Scope  NumInputPorts=2
  mapping_factor : Gain  Gain=64.0 / 50.0
  throttle_command : Outport
  wires:
  mapping_factor/1 -> Data Type Conversion/1
  measured_height/1 -> Sum2/2, Z_error/1
  z_desired/1 -> Z_error/2, Sum2/1
  Sum2/1 -> To Workspace1/1, If/1
  Merge/1 -> Moving Average/1
  Data Type Conversion/1 -> throttle_command/1
  If/1 -> If Action Subsystem/Action
  If/2 -> If Action Subsystem1/Action
  If/3 -> If Action Subsystem2/Action
  Constant/1 -> If Action Subsystem/1(In1)
  Constant1/1 -> If Action Subsystem1/1(In1)
  Constant2/1 -> If Action Subsystem2/1(In1)
  If Action Subsystem1/1(Out1) -> Merge/2
  If Action Subsystem/1(Out1) -> Merge/1
  If Action Subsystem2/1(Out1) -> Merge/3
  Moving Average/1 -> To Workspace/1, Z_command/1, mapping_factor/1

== system guidance_fuzzy_alt/Subsystem5 ==
  height : Inport
  vx : Inport  Port=2
  vy : Inport  Port=3
  Demux1 : Demux  Outputs=2
  If Action Subsystem2 : Subsystem  TreatAsAtomicUnit=on
  If Action Subsystem3 : Subsystem  TreatAsAtomicUnit=on
  Merge1 : Merge
  Mux : Mux  Inputs=2
  Mux1 : Mux  Inputs=2
  ground_detection_condition : If  IfExpression=u1 < 0.0
  zero_velocity : Constant  Value=0
  vx_out : Outport
  vy_out : Outport  Port=2
  wires:
  vy/1 -> Mux1/2
  vx/1 -> Mux1/1
  height/1 -> ground_detection_condition/1
  Demux1/1 -> vx_out/1
  zero_velocity/1 -> Mux/2, Mux/1
  Demux1/2 -> vy_out/1
  ground_detection_condition/1 -> If Action Subsystem2/Action
  If Action Subsystem3/1(Out1) -> Merge1/2
  Merge1/1 -> Demux1/1
  Mux1/1 -> If Action Subsystem3/1(In1)
  ground_detection_condition/2 -> If Action Subsystem3/Action
  If Action Subsystem2/1(Out1) -> Merge1/1
  Mux/1 -> If Action Subsystem2/1(In1)

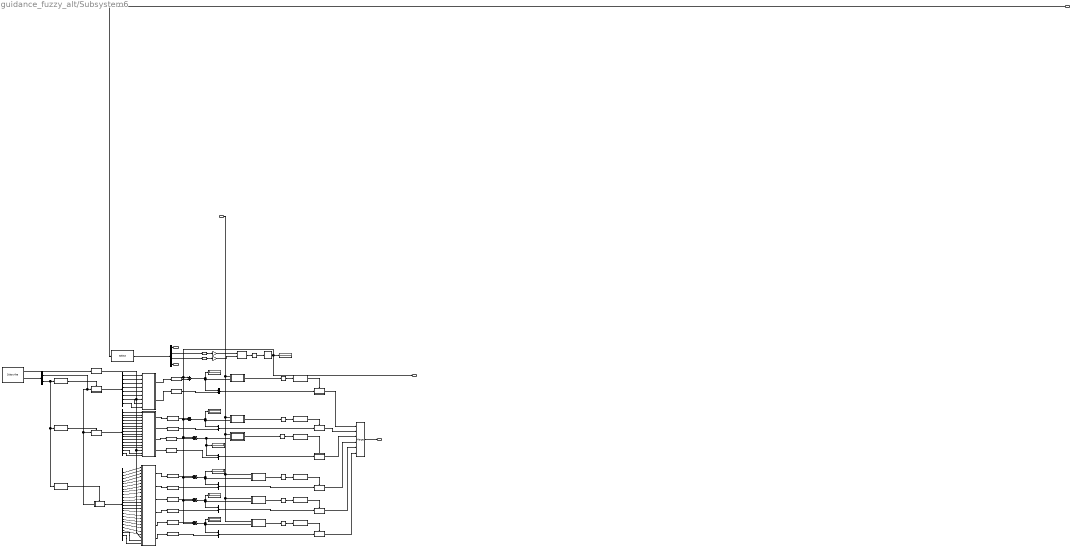
== system guidance_fuzzy_alt/Subsystem6 ==
  In1 : Inport
  In2 : Inport  Port=2
  Abs{,1..5} (6 alike) : Abs
  Bus Selector : BusSelector  OutputSignals=Data,Data_SL_Info.CurrentLength
  Data Type Conversion{,1..2,7..16} (13 alike) : DataTypeConversion  OutDataTypeStr=double
  Data Type Conversion5 : DataTypeConversion  OutDataTypeStr=single
  Data Type Conversion6 : DataTypeConversion  OutDataTypeStr=single
  Demux2 : Demux  Outputs=8
  Demux3 : Demux  Outputs=16
  Demux4 : Demux  Outputs=24
  Demux5 : Demux
  Display{1,3,5,14..17} (7 alike) : Display
  Gain : Gain  Gain=-1
  Gain1 : Gain  Gain=-1
  If Action Subsystem1 : Subsystem  TreatAsAtomicUnit=on
  If Action Subsystem10 : Subsystem  TreatAsAtomicUnit=on
  If Action Subsystem11 : Subsystem  TreatAsAtomicUnit=on
  If Action Subsystem12 : Subsystem  TreatAsAtomicUnit=on
  If Action Subsystem13 : Subsystem  TreatAsAtomicUnit=on
  If Action Subsystem14 : Subsystem  TreatAsAtomicUnit=on
  If Action Subsystem15 : Subsystem  TreatAsAtomicUnit=on
  If Action Subsystem4 : Subsystem  TreatAsAtomicUnit=on
  If Action Subsystem5 : Subsystem  TreatAsAtomicUnit=on
  If{2..4,8..10} (6 alike) : If  IfExpression=u1 < 20  ShowElse=off
  If5 : If  IfExpression=u1 ==8  ShowElse=off
  If6 : If  IfExpression=u1 ==16  ShowElse=off
  If7 : If  IfExpression=u1 ==24  ShowElse=off
  Merge5 : Merge  Inputs=6
  Moving Average2 : dspstat3/Moving Average  Method=Sliding window  SpecifyWindowLength=on  WindowLength=20  ForgettingFactor=0.9  SimulateUsing=Code generation
  Mux{,1..2,5..7} (6 alike) : Mux  Inputs=2
  Radians to Degrees : simulink_extras/Transformations/Radians to Degrees
  Selector3 : Selector  InputPortWidth=26  IndexOptions=Index vector (dialog)  Indices=[3 14 15 16]  OutputSizes=1
  Subscribe2 : robotlib/Subscribe  SourceLibraryInfo=This block requires Robotics System Toolbox  topicSource=Select from ROS network  topic=/quadrotor_1/line_data  messageType=std_msgs/Int16MultiArray  sampleTime=-1  messageQueueLength=1
      settings: SourceProductBaseCode=RO
  Subsystem1 : Subsystem
  Subsystem3 : Subsystem
  Subsystem4 : Subsystem
  Sum{1..6} (6 alike) : Sum
  Trigonometric Function : Trigonometry  Operator=atan2
  optimize_error_psi(deg) : Subsystem
  optimize_error_psi(deg)1 : Subsystem
  optimize_error_psi(deg)2 : Subsystem
  optimize_error_psi(deg)4 : Subsystem
  optimize_error_psi(deg)5 : Subsystem
  optimize_error_psi(deg)6 : Subsystem
  Out1 : Outport
  Out2 : Outport  Port=2
  Out3 : Outport  Port=3
  Out4 : Outport  Port=4
  wires:
  If Action Subsystem11/1(Out1) -> Demux3/1
  optimize_error_psi(deg)/1(Out1) -> Abs/1
  Data Type Conversion5/1 -> Gain1/1
  Sum5/1 -> Display17/1, Mux2/1, optimize_error_psi(deg)2/2(psi2)
  If Action Subsystem10/1(Out1) -> Demux2/1
  Abs/1 -> If8/1
  If6/1 -> If Action Subsystem11/Action
  Selector3/1 -> Demux5/1
  Bus Selector/2 -> If7/1, If6/1, If5/1  "<CurrentLength>"
  Sum4/1 -> Display16/1, Mux1/1, optimize_error_psi(deg)1/2(psi2)
  Demux5/2 -> Data Type Conversion6/1
  Trigonometric Function/1 -> Radians to Degrees/1
  Data Type Conversion9/1 -> Sum5/2
  Data Type Conversion11/1 -> Sum3/2
  optimize_error_psi(deg)2/1(Out1) -> Abs2/1
  If Action Subsystem14/1(Out1) -> Merge5/2
  Gain/1 -> Trigonometric Function/1
  Subsystem3/4(distance2) -> Data Type Conversion10/1
  Subsystem3/1(angle) -> Data Type Conversion7/1
  Radians to Degrees/1 -> Moving Average2/1
  If Action Subsystem12/1(Out1) -> Demux4/1
  optimize_error_psi(deg)1/1(Out1) -> Abs1/1
  Data Type Conversion6/1 -> Gain/1
  Abs1/1 -> If9/1
  Mux2/1 -> If Action Subsystem15/1(In1)
  Subsystem3/2(distance1) -> Data Type Conversion8/1
  If5/1 -> If Action Subsystem10/Action
  Subscribe2/2 -> Bus Selector/1
  Merge5/1 -> Out4/1
  If7/1 -> If Action Subsystem12/Action
  Gain1/1 -> Trigonometric Function/2
  Bus Selector/1 -> If Action Subsystem11/1(In1), If Action Subsystem12/1(In1), If Action Subsystem10/1(In1)  "<Data>"
  Demux5/4 -> Out2/1
  Demux5/1 -> Out1/1
  Demux3/7 -> Subsystem3/7(xc)
  Demux3/8 -> Subsystem3/8(yc)
  Demux3/9 -> Subsystem3/9(x2)
  Demux3/10 -> Subsystem3/10(y2)
  Demux3/11 -> Subsystem3/11(x3)
  Demux3/12 -> Subsystem3/12(y3)
  Demux3/13 -> Subsystem3/13(xi1)
  Demux3/14 -> Subsystem3/14(yi1)
  Demux3/15 -> Subsystem3/16(xc1)
  Demux3/16 -> Subsystem3/17(yc1)
  Demux4/1 -> Subsystem4/1(x0)
  Demux4/10 -> Subsystem4/10(y2)
  Demux4/2 -> Subsystem4/2(y0)
  Demux4/3 -> Subsystem4/3(x1)
  Demux4/4 -> Subsystem4/4(y1)
  Demux4/5 -> Subsystem4/5(xi)
  Demux4/6 -> Subsystem4/6(yi)
  Demux4/7 -> Subsystem4/7(xc)
  Demux4/17 -> Subsystem4/17(x4)
  Demux4/8 -> Subsystem4/8(yc)
  Demux4/9 -> Subsystem4/9(x2)
  Demux4/11 -> Subsystem4/11(x3)
  Demux4/12 -> Subsystem4/12(y3)
  Demux4/13 -> Subsystem4/13(xi1)
  Demux4/14 -> Subsystem4/14(yi1)
  Demux4/15 -> Subsystem4/15(xc1)
  Demux4/16 -> Subsystem4/16(yc1)
  Demux4/18 -> Subsystem4/18(y4)
  Demux4/19 -> Subsystem4/19(x5)
  Demux4/20 -> Subsystem4/20(y5)
  Demux4/21 -> Subsystem4/21(xi2)
  Demux4/22 -> Subsystem4/22(yi2)
  Demux4/23 -> Subsystem4/24(xc2)
  Demux4/24 -> Subsystem4/25(yc2)
  Subsystem1/1(angle) -> Data Type Conversion11/1
  Demux3/3 -> Subsystem3/3(x1)
  Demux3/2 -> Subsystem3/2(y0)
  Demux3/1 -> Subsystem3/1(x0)
  Demux2/7 -> Subsystem1/8(xc)
  Demux2/8 -> Subsystem1/9(yc)
  Demux2/1 -> Subsystem1/1(x0)
  Demux2/2 -> Subsystem1/2(y0)
  Demux2/3 -> Subsystem1/3(x1)
  Demux2/4 -> Subsystem1/4(y1)
  Demux2/5 -> Subsystem1/5(xi)
  Demux2/6 -> Subsystem1/6(yi)
  Mux7/1 -> If Action Subsystem5/1(In1)
  Subsystem4/4(distance2) -> Data Type Conversion14/1
  Subsystem4/3(angle1) -> Data Type Conversion13/1
  Data Type Conversion7/1 -> Sum4/1
  If10/1 -> If Action Subsystem15/Action
  If9/1 -> If Action Subsystem14/Action
  If8/1 -> If Action Subsystem13/Action
  If Action Subsystem13/1(Out1) -> Merge5/1
  Data Type Conversion8/1 -> Mux1/2
  Mux/1 -> If Action Subsystem13/1(In1)
  Subsystem3/3(angle1) -> Data Type Conversion9/1
  Data Type Conversion12/1 -> Mux/2
  Demux5/3 -> Data Type Conversion5/1
  If Action Subsystem15/1(Out1) -> Merge5/3
  Data Type Conversion10/1 -> Mux2/2
  Sum3/1 -> Display14/1, Mux/1, optimize_error_psi(deg)/2(psi2)
  Mux1/1 -> If Action Subsystem14/1(In1)
  Abs2/1 -> If10/1
  Subsystem1/2(distance1) -> Data Type Conversion12/1
  optimize_error_psi(deg)4/1(Out1) -> Abs3/1
  Data Type Conversion1/1 -> Sum1/1
  Subsystem4/2(distance1) -> Data Type Conversion2/1
  Abs3/1 -> If2/1
  Subsystem4/1(angle) -> Data Type Conversion1/1
  If Action Subsystem1/1(Out1) -> Merge5/4
  Sum1/1 -> Display1/1, Mux5/1, optimize_error_psi(deg)4/2(psi2)
  If2/1 -> If Action Subsystem1/Action
  Mux5/1 -> If Action Subsystem1/1(In1)
  Data Type Conversion2/1 -> Mux5/2
  Mux6/1 -> If Action Subsystem4/1(In1)
  If3/1 -> If Action Subsystem4/Action
  If Action Subsystem4/1(Out1) -> Merge5/5
  Data Type Conversion13/1 -> Sum2/1
  Sum2/1 -> Display3/1, Mux6/1, optimize_error_psi(deg)5/2(psi2)
  Moving Average2/1 -> Sum6/2, Sum2/2, Sum1/2, Sum5/1, Sum4/2, Sum3/1, Out3/1, Display15/1
  optimize_error_psi(deg)5/1(Out1) -> Abs4/1
  Data Type Conversion14/1 -> Mux6/2
  Abs4/1 -> If3/1
  Data Type Conversion/1 -> Subsystem1/7(isnew), Subsystem4/23(isnew2), Subsystem3/15(isnew)
  Abs5/1 -> If4/1
  Subsystem4/6(distance3) -> Data Type Conversion16/1
  Subscribe2/1 -> Data Type Conversion/1
  Subsystem4/5(angle2) -> Data Type Conversion15/1
  Sum6/1 -> Display5/1, Mux7/1, optimize_error_psi(deg)6/2(psi2)
  Data Type Conversion16/1 -> Mux7/2
  optimize_error_psi(deg)6/1(Out1) -> Abs5/1
  Data Type Conversion15/1 -> Sum6/1
  If Action Subsystem5/1(Out1) -> Merge5/6
  If4/1 -> If Action Subsystem5/Action
  Demux3/6 -> Subsystem3/6(yi)
  Demux3/4 -> Subsystem3/4(y1)
  Demux3/5 -> Subsystem3/5(xi)
  In2/1 -> optimize_error_psi(deg)6/1(psi1), optimize_error_psi(deg)5/1(psi1), optimize_error_psi(deg)4/1(psi1), optimize_error_psi(deg)2/1(psi1), optimize_error_psi(deg)1/1(psi1), optimize_error_psi(deg)/1(psi1)
  In1/1 -> Selector3/1

== system guidance_fuzzy_alt/attitude_failsafe ==
  attitude : Inport
  user_arm_command : Inport  Port=2
  Abs : Abs  OutDataTypeStr=single
  Constant : Constant  Value=0
  Data Store Read : DataStoreRead  DataStoreName=kill
  Demux7 : Demux  Outputs=2
  Display1 : Display
  If : If  NumInputs=2  IfExpression=u1 < 40 & u2 < 40
  If Action Subsystem : Subsystem  TreatAsAtomicUnit=on
  If Action Subsystem1 : Subsystem  TreatAsAtomicUnit=on
  If Action Subsystem2 : Subsystem  TreatAsAtomicUnit=on
  If Action Subsystem3 : Subsystem  TreatAsAtomicUnit=on
  If Action Subsystem4 : Subsystem  TreatAsAtomicUnit=on
  If1 : If  IfExpression=u1 == 1
  If2 : If  IfExpression=u1 == 0  ShowElse=off
  Merge : Merge
  arm_command : Outport
  wires:
  attitude/1 -> Abs/1
  Demux7/1 -> If/1
  Demux7/2 -> If/2
  If/2 -> If Action Subsystem1/Action
  If/1 -> If Action Subsystem/Action
  Merge/1 -> arm_command/1
  Abs/1 -> Demux7/1, Display1/1
  Data Store Read/1 -> If1/1
  If1/1 -> If Action Subsystem2/Action
  If1/2 -> If Action Subsystem3/Action
  user_arm_command/1 -> If2/1, If Action Subsystem3/1(In1)
  Constant/1 -> If Action Subsystem2/1(In1)
  If Action Subsystem2/1(Out1) -> Merge/1
  If Action Subsystem3/1(Out1) -> Merge/2
  If2/1 -> If Action Subsystem4/Action

== system guidance_fuzzy_alt/check_arm_status ==
  arm : Inport
  command : Inport  Port=2
  motors_on : Inport  Port=3
  Constant4 : Constant  Value=[0 0 0 0 127]
  Constant5 : Constant  Value=[0 0 0 0 127]
  If : If  NumInputs=2  IfExpression=u1 & ~u2  ElseIfExpressions=~u1 & u2
  If Action Subsystem1 : Subsystem  TreatAsAtomicUnit=on
  If Action Subsystem2 : Subsystem  TreatAsAtomicUnit=on
  If Action Subsystem3 : Subsystem  TreatAsAtomicUnit=on
  Merge : Merge  Inputs=3
  Out : Outport
  wires:
  If/1 -> If Action Subsystem1/Action
  Constant4/1 -> If Action Subsystem2/1(In1)
  If/3 -> If Action Subsystem3/Action
  Constant5/1 -> If Action Subsystem1/1(In1)
  If/2 -> If Action Subsystem2/Action
  If Action Subsystem2/1(Out1) -> Merge/2
  motors_on/1 -> If/2
  command/1 -> If Action Subsystem3/1(In1)
  If Action Subsystem1/1(Out1) -> Merge/1
  If Action Subsystem3/1(Out1) -> Merge/3
  arm/1 -> If/1
  Merge/1 -> Out/1

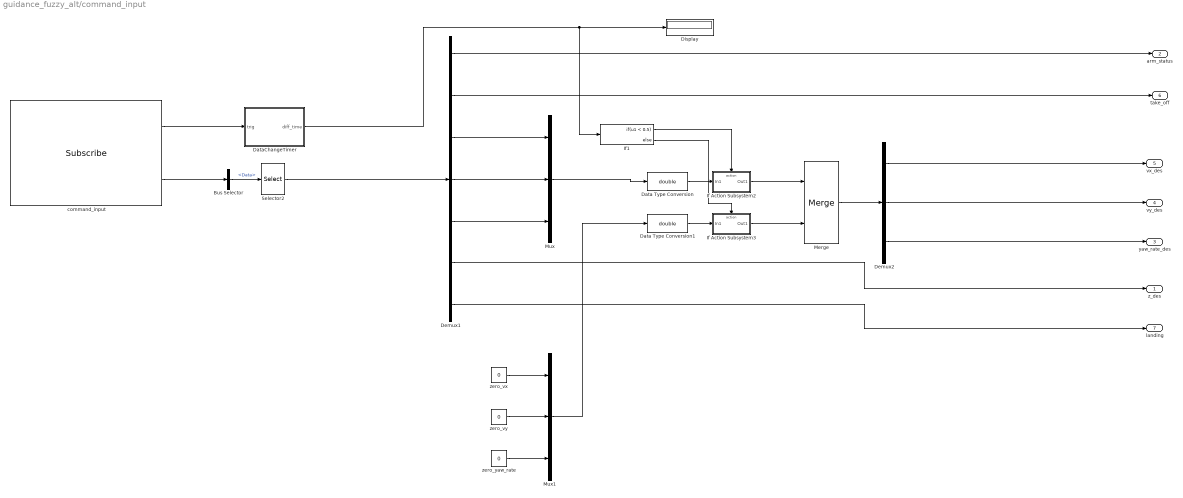
== system guidance_fuzzy_alt/command_input ==
  Bus Selector : BusSelector  OutputSignals=Data
  Data Type Conversion : DataTypeConversion  OutDataTypeStr=double
  Data Type Conversion1 : DataTypeConversion  OutDataTypeStr=double
  DataChangeTimer : Subsystem
  Demux1 : Demux  Outputs=7
  Demux2 : Demux  Outputs=3
  Display : Display
  If Action Subsystem2 : Subsystem  TreatAsAtomicUnit=on
  If Action Subsystem3 : Subsystem  TreatAsAtomicUnit=on
  If1 : If  IfExpression=u1 < 0.5
  Merge : Merge
  Mux : Mux  Inputs=3
  Mux1 : Mux  Inputs=3
  Selector2 : Selector  InputPortWidth=128  IndexOptions=Index vector (dialog)  Indices=[1 2 3 4 5 6 7]  OutputSizes=1
  command_input : robotlib/Subscribe  SourceLibraryInfo=This block requires Robotics System Toolbox  topicSource=Specify your own  topic=/quadrotor_1/road_following_cmd  messageType=std_msgs/Float32MultiArray  sampleTime=-1  messageQueueLength=1
      settings: SourceProductBaseCode=RO
  zero_vx : Constant  Value=0
  zero_vy : Constant  Value=0
  zero_yaw_rate : Constant  Value=0
  z_des : Outport
  arm_status : Outport  Port=2
  yaw_rate_des : Outport  Port=3
  vy_des : Outport  Port=4
  vx_des : Outport  Port=5
  take_off : Outport  Port=6
  landing : Outport  Port=7
  wires:
  DataChangeTimer/1(diff_time) -> If1/1, Display/1
  If1/2 -> If Action Subsystem3/Action
  Demux1/5 -> Mux/3
  Demux1/1 -> arm_status/1
  Demux2/1 -> vx_des/1
  If1/1 -> If Action Subsystem2/Action
  Demux1/4 -> Mux/2
  command_input/1 -> DataChangeTimer/1(trig)
  Mux/1 -> Data Type Conversion/1
  command_input/2 -> Bus Selector/1
  Bus Selector/1 -> Selector2/1  "<Data>"
  Demux1/2 -> take_off/1
  Demux2/2 -> vy_des/1
  Demux1/6 -> z_des/1
  Demux2/3 -> yaw_rate_des/1
  Selector2/1 -> Demux1/1
  zero_yaw_rate/1 -> Mux1/3
  zero_vx/1 -> Mux1/1
  Mux1/1 -> Data Type Conversion1/1
  zero_vy/1 -> Mux1/2
  Demux1/3 -> Mux/1
  Merge/1 -> Demux2/1
  Demux1/7 -> landing/1
  If Action Subsystem2/1(Out1) -> Merge/1
  If Action Subsystem3/1(Out1) -> Merge/2
  Data Type Conversion/1 -> If Action Subsystem2/1(In1)
  Data Type Conversion1/1 -> If Action Subsystem3/1(In1)

== system guidance_fuzzy_alt/command_output ==
  command : Inport
  Assignment : Assignment  DiagnosticForDimensions=Warning  IndexOptions=Index vector (dialog)  Indices=[1 2 3 4 5]  OutputSizes=1
  Blank Message : robotlib/Blank Message  SourceLibraryInfo=This block requires Robotics System Toolbox  messageType=std_msgs/Int16MultiArray  SampleTime=inf
      settings: SourceProductBaseCode=RO
  Bus Assignment : BusAssignment  AssignedSignals=Data,Data_SL_Info.CurrentLength
  Constant : Constant  Value=[1:1:128]
  Constant1 : Constant  Value=5
  Data Type Conversion : DataTypeConversion  OutDataTypeStr=double
  Data Type Conversion1 : DataTypeConversion  OutDataTypeStr=uint32
  Data Type Conversion2 : DataTypeConversion  OutDataTypeStr=int16
  "command_output " : robotlib/Publish  SourceLibraryInfo=This block requires Robotics System Toolbox  topicSource=Select from ROS network  topic=/quadrotor_1/rpyt_command  messageType=std_msgs/Int16MultiArray  messageQueueLength=1
      settings: SourceProductBaseCode=RO
  wires:
  Constant1/1 -> Data Type Conversion1/1
  Data Type Conversion1/1 -> Bus Assignment/3
  Bus Assignment/1 -> "command_output "/1
  Data Type Conversion2/1 -> Bus Assignment/2
  Assignment/1 -> Data Type Conversion2/1
  Blank Message/1 -> Bus Assignment/1
  Data Type Conversion/1 -> Assignment/2
  command/1 -> Data Type Conversion/1
  Constant/1 -> Assignment/1

== system guidance_fuzzy_alt/compensate_angular_velocity_effect_on_of ==
  vx : Inport
  vy : Inport  Port=2
  p : Inport  Port=3
  q : Inport  Port=4
  Sum : Sum  Inputs=|+-
  Sum1 : Sum  Inputs=|+-
  p_correction_factor : Gain  Gain=0.7
  q_correction_factor : Gain  Gain=0.7
  corrected_vx : Outport
  corrected_vy : Outport  Port=2
  wires:
  vx/1 -> Sum/1
  vy/1 -> Sum1/1
  q/1 -> q_correction_factor/1
  p/1 -> p_correction_factor/1
  Sum1/1 -> corrected_vy/1
  Sum/1 -> corrected_vx/1
  p_correction_factor/1 -> Sum1/2
  q_correction_factor/1 -> Sum/2

== system guidance_fuzzy_alt/data_input  ==
  Bus Selector : BusSelector  OutputSignals=Data
  Bus Selector1 : BusSelector  OutputSignals=Data
  Bus Selector2 : BusSelector  OutputSignals=Data
  Demux : Demux  Outputs=2
  Selector : Selector  InputPortWidth=128  IndexOptions=Index vector (dialog)  Indices=[1 2 3 4 5 6]  OutputSizes=1
  Selector1 : Selector  InputPortWidth=128  IndexOptions=Index vector (dialog)  Indices=[1 2 3 4 5 6 7 8 9 10 11 12 13 14 15 16 17 18]  OutputSizes=1
  Selector2 : Selector  InputPortWidth=128  IndexOptions=Index vector (dialog)  Indices=[1 2]  OutputSizes=1
  Subscribe : robotlib/Subscribe  SourceLibraryInfo=This block requires Robotics System Toolbox  topicSource=Select from ROS network  topic=/quadrotor_1/nav  messageType=std_msgs/Float32MultiArray  sampleTime=-1  messageQueueLength=1
      settings: SourceProductBaseCode=RO
  Subscribe1 : robotlib/Subscribe  SourceLibraryInfo=This block requires Robotics System Toolbox  topicSource=Select from ROS network  topic=/quadrotor_1/optical_flow  messageType=std_msgs/Float32MultiArray  sampleTime=-1  messageQueueLength=1
      settings: SourceProductBaseCode=RO
  Subscribe2 : robotlib/Subscribe  SourceLibraryInfo=This block requires Robotics System Toolbox  topicSource=Select from ROS network  topic=/quadrotor_1/sensor_data  messageType=std_msgs/Float32MultiArray  sampleTime=-1  messageQueueLength=1
      settings: SourceProductBaseCode=RO
  Terminator : Terminator
  Terminator1 : Terminator
  Terminator2 : Terminator
  Vector Concatenate : Concatenate  NumInputs=4
  data : Outport
  wires:
  Subscribe/1 -> Terminator/1
  Selector/1 -> Vector Concatenate/2
  Subscribe2/1 -> Terminator1/1
  Subscribe2/2 -> Bus Selector1/1
  Subscribe/2 -> Bus Selector/1
  Bus Selector/1 -> Selector/1  "<Data>"
  Bus Selector1/1 -> Selector1/1  "<Data>"
  Selector1/1 -> Vector Concatenate/1
  Vector Concatenate/1 -> data/1
  Subscribe1/2 -> Bus Selector2/1
  Subscribe1/1 -> Terminator2/1
  Bus Selector2/1 -> Selector2/1  "<Data>"
  Selector2/1 -> Demux/1
  Demux/1 -> Vector Concatenate/3
  Demux/2 -> Vector Concatenate/4

== system guidance_fuzzy_alt/manual_control ==
  Constant : Constant  Value=[mode throttle roll pitch yaw]
  commands : Outport
  wires:
  Constant/1 -> commands/1

== system guidance_fuzzy_alt/manual_throttle ==
  mode1 : Constant  Value=th
  Out1 : Outport
  wires:
  mode1/1 -> Out1/1

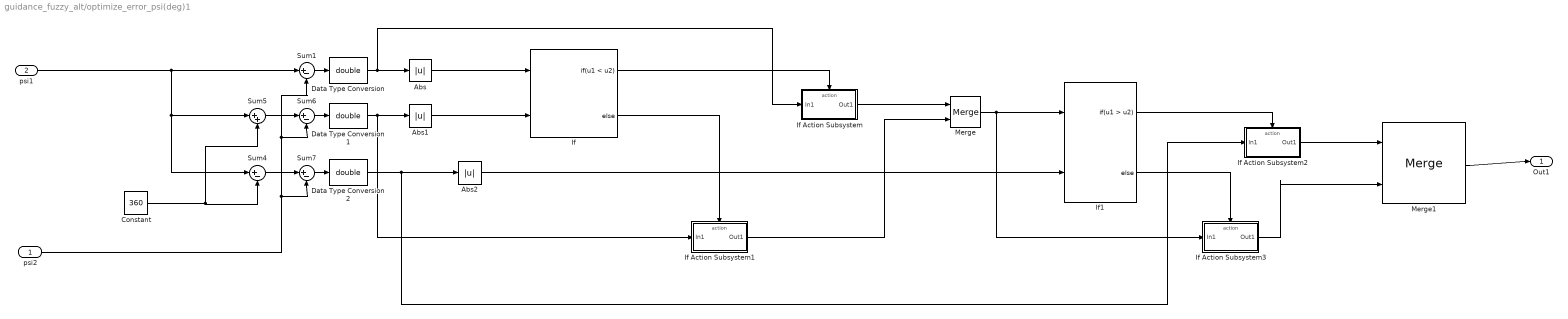
== system guidance_fuzzy_alt/optimize_error_psi(deg)1 ==
  psi2 : Inport
  psi1 : Inport  Port=2
  Abs : Abs
  Abs1 : Abs
  Abs2 : Abs
  Constant : Constant  Value=360
  Data Type Conversion : DataTypeConversion  OutDataTypeStr=double
  Data Type Conversion1 : DataTypeConversion  OutDataTypeStr=double
  Data Type Conversion2 : DataTypeConversion  OutDataTypeStr=double
  If : If  NumInputs=2  IfExpression=u1 < u2
  If Action Subsystem : Subsystem  TreatAsAtomicUnit=on
  If Action Subsystem1 : Subsystem  TreatAsAtomicUnit=on
  If Action Subsystem2 : Subsystem  TreatAsAtomicUnit=on
  If Action Subsystem3 : Subsystem  TreatAsAtomicUnit=on
  If1 : If  NumInputs=2  IfExpression=u1 > u2
  Merge : Merge
  Merge1 : Merge
  Sum{1,4,6..7} (4 alike) : Sum  Inputs=|+-
  Sum5 : Sum  Inputs=|++
  Out1 : Outport
  wires:
  Data Type Conversion2/1 -> Abs2/1, If Action Subsystem2/1(In1)
  Data Type Conversion1/1 -> Abs1/1, If Action Subsystem1/1(In1)
  Data Type Conversion/1 -> If Action Subsystem/1(In1), Abs/1
  Sum5/1 -> Sum6/1
  If Action Subsystem1/1(Out1) -> Merge/2
  Sum6/1 -> Data Type Conversion1/1
  Abs/1 -> If/1
  If Action Subsystem/1(Out1) -> Merge/1
  If Action Subsystem2/1(Out1) -> Merge1/1
  Sum7/1 -> Data Type Conversion2/1
  If/2 -> If Action Subsystem1/Action
  If/1 -> If Action Subsystem/Action
  Sum1/1 -> Data Type Conversion/1
  Abs2/1 -> If1/2
  Merge/1 -> If1/1, If Action Subsystem3/1(In1)
  Merge1/1 -> Out1/1
  Abs1/1 -> If/2
  Sum4/1 -> Sum7/1
  Constant/1 -> Sum4/2, Sum5/2
  If1/2 -> If Action Subsystem3/Action
  If Action Subsystem3/1(Out1) -> Merge1/2
  If1/1 -> If Action Subsystem2/Action
  psi2/1 -> Sum1/2, Sum6/2, Sum7/2
  psi1/1 -> Sum4/1, Sum5/1, Sum1/1

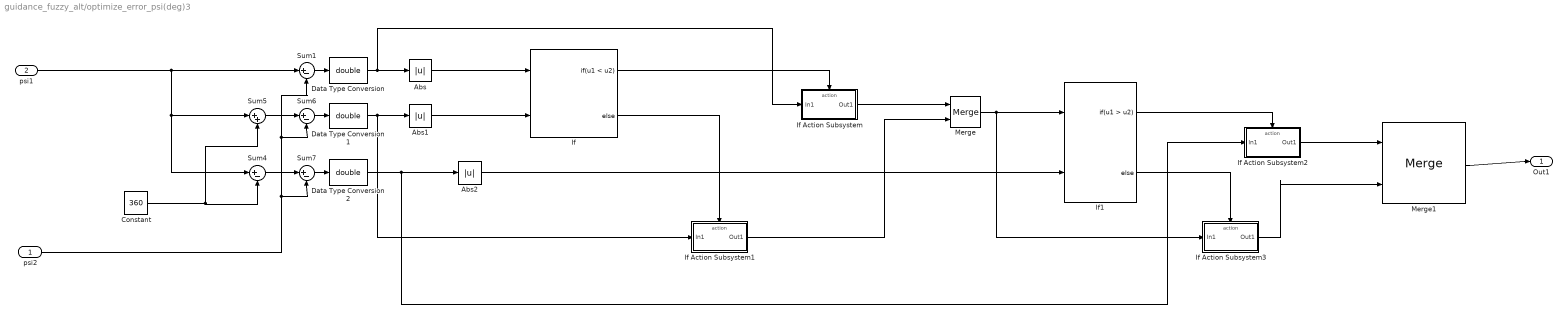
== system guidance_fuzzy_alt/optimize_error_psi(deg)3 ==
  psi2 : Inport
  psi1 : Inport  Port=2
  Abs : Abs
  Abs1 : Abs
  Abs2 : Abs
  Constant : Constant  Value=360
  Data Type Conversion : DataTypeConversion  OutDataTypeStr=double
  Data Type Conversion1 : DataTypeConversion  OutDataTypeStr=double
  Data Type Conversion2 : DataTypeConversion  OutDataTypeStr=double
  If : If  NumInputs=2  IfExpression=u1 < u2
  If Action Subsystem : Subsystem  TreatAsAtomicUnit=on
  If Action Subsystem1 : Subsystem  TreatAsAtomicUnit=on
  If Action Subsystem2 : Subsystem  TreatAsAtomicUnit=on
  If Action Subsystem3 : Subsystem  TreatAsAtomicUnit=on
  If1 : If  NumInputs=2  IfExpression=u1 > u2
  Merge : Merge
  Merge1 : Merge
  Sum{1,4,6..7} (4 alike) : Sum  Inputs=|+-
  Sum5 : Sum  Inputs=|++
  Out1 : Outport
  wires:
  psi1/1 -> Sum1/1, Sum5/1, Sum4/1
  psi2/1 -> Sum7/2, Sum6/2, Sum1/2
  If1/1 -> If Action Subsystem2/Action
  If Action Subsystem3/1(Out1) -> Merge1/2
  If1/2 -> If Action Subsystem3/Action
  Constant/1 -> Sum5/2, Sum4/2
  Sum4/1 -> Sum7/1
  Abs1/1 -> If/2
  Merge1/1 -> Out1/1
  Merge/1 -> If Action Subsystem3/1(In1), If1/1
  Abs2/1 -> If1/2
  Sum1/1 -> Data Type Conversion/1
  If/1 -> If Action Subsystem/Action
  If/2 -> If Action Subsystem1/Action
  Sum7/1 -> Data Type Conversion2/1
  If Action Subsystem2/1(Out1) -> Merge1/1
  If Action Subsystem/1(Out1) -> Merge/1
  Abs/1 -> If/1
  Sum6/1 -> Data Type Conversion1/1
  If Action Subsystem1/1(Out1) -> Merge/2
  Sum5/1 -> Sum6/1
  Data Type Conversion/1 -> Abs/1, If Action Subsystem/1(In1)
  Data Type Conversion1/1 -> If Action Subsystem1/1(In1), Abs1/1
  Data Type Conversion2/1 -> If Action Subsystem2/1(In1), Abs2/1
